simulink model "xpctankpanel"  (Simulink 6.0)
settings: Solver=FixedStepDiscrete  StartTime=0.0  StopTime=inf  RelTol=1e-3
libraries: xpclib x8, dnglibv1 x7
settings Model: Creator=mvetsch  LastModifiedBy=shaishaa  ExtModeTrigMode=oneshot  ExtModeArmWhenConnect=off  ProdHWDeviceType=Specified
settings DataIOCC: LimitDataPoints=off  SignalLoggingName=logsOut
settings OptimizationCC: BlockReduction=off  BooleanDataType=off  MultiInstanced=off
settings FormatCC: IgnoreBidirectionalLines=off
settings HardwareCC: ProdHWDeviceType=Specified
settings CodeAppCC: FileBanners=off  CustomSymbols=off
settings GRTTargetCC: TargetFcnLib=iso_c_tmw.mat  IsERTTarget=off

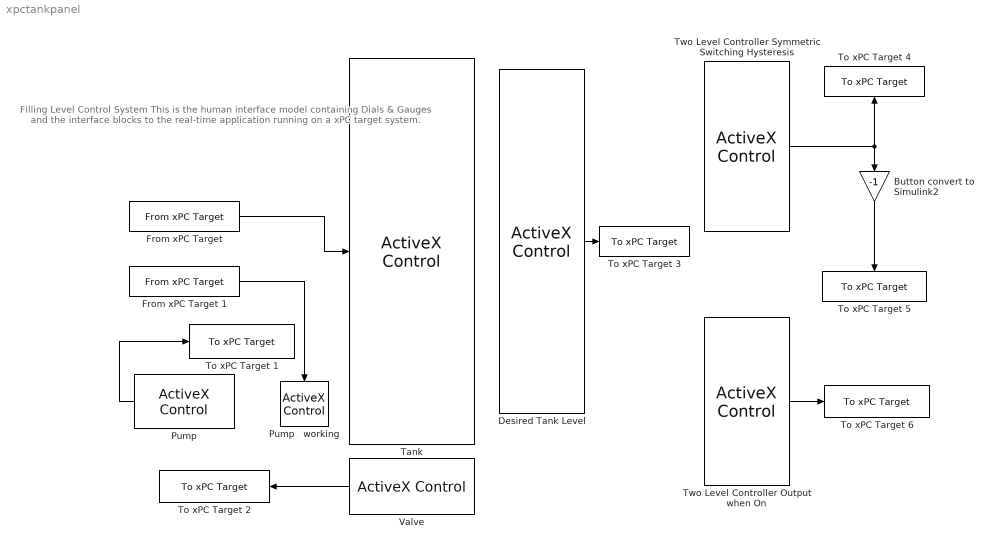
== system xpctankpanel ==
  note: Filling Level Control System
      | This is the human interface model containing
      | Dials & Gauges and the interface blocks
      | to the real-time application running on a
      | xPC target system.
  "  Pump   working" : dnglibv1/ActiveX Control  Orientation=down  progid=MWLED.ledctrl.1  connect=input  input=Value  init=hActx.configuration='LED\Individual\Red Circular Bitmap';hActx.value=1;hActx.Mode=0;hActx.MouseControl=0;  inblock=on  border=off  dialOut=0  updateParam=0
  Button convert to Simulink2 : Gain  Orientation=down  Gain=-1  SaturateOnIntegerOverflow=on
  Desired Tank Level : dnglibv1/ActiveX Control  progid=mwslider.sliderctrl.1  connect=output  output=Value  dialOutEvent=Slide Change  init=hActx.configuration='Slider\Big Numbers';  inblock=on  border=off  dialOut=0  updateParam=0
  "From xPC Target  " : xpclib/Misc./From xPC Target   appname=xpctank  blockpath=TankLevel  ts=1
  From xPC Target 1 : xpclib/Misc./From xPC Target   appname=xpctank  blockpath=ControlValue  ts=1
  Pump : dnglibv1/ActiveX Control  Orientation=left  progid=mwtoggle.togglectrl.1  connect=output  output=Value  dialOutEvent=Click  inblock=on  border=off  dialOut=0  updateParam=0
  Tank : dnglibv1/ActiveX Control  progid=mwslider.sliderctrl.1  connect=input  input=Value  init=hActx.configuration='Slider\Water Tank';  inblock=on  border=off  dialOut=0  updateParam=0
  To xPC Target 1 : xpclib/Misc./To xPC Target   appname=xpctank  blockpath=PumpSwitch  paramname=Value
  To xPC Target 2 : xpclib/Misc./To xPC Target   Orientation=left  appname=xpctank  blockpath=ValveSwitch  paramname=Value
  To xPC Target 3 : xpclib/Misc./To xPC Target   appname=xpctank  blockpath=SetPoint  paramname=Value
  To xPC Target 4 : xpclib/Misc./To xPC Target   Orientation=up  appname=xpctank  blockpath=Controller  paramname=OnSwitchValue
  To xPC Target 5 : xpclib/Misc./To xPC Target   Orientation=down  appname=xpctank  blockpath=Controller  paramname=OffSwitchValue
  To xPC Target 6 : xpclib/Misc./To xPC Target   appname=xpctank  blockpath=Controller  paramname=OnOutputValue
  Two Level Controller Output when On : dnglibv1/ActiveX Control  progid=mwslider.sliderctrl.1  connect=output  output=Value  dialOutEvent=Slide Change  init=hActx.configuration='Slider\Big Numbers';  inblock=on  border=off  dialOut=0  updateParam=0
  Two Level Controller Symmetric Switching Hysteresis : dnglibv1/ActiveX Control  progid=mwslider.sliderctrl.1  connect=output  output=Value  dialOutEvent=Slide Change  init=hActx.configuration='Slider\Big Numbers';  inblock=on  border=off  dialOut=0  updateParam=0
  Valve : dnglibv1/ActiveX Control  Orientation=left  progid=mwtoggle.togglectrl.1  connect=output  output=Value  dialOutEvent=Click  inblock=on  border=off  dialOut=0  updateParam=0
  wires:
  Desired Tank Level/1 -> To xPC Target 3/1
  Valve/1 -> To xPC Target 2/1
  "From xPC Target  "/1 -> Tank/1
  Two Level Controller Output when On/1 -> To xPC Target 6/1
  Button convert to Simulink2/1 -> To xPC Target 5/1
  Two Level Controller Symmetric Switching Hysteresis/1 -> To xPC Target 4/1, Button convert to Simulink2/1
  From xPC Target 1/1 -> "  Pump   working"/1
  Pump/1 -> To xPC Target 1/1
